simulink model "trans"  (R2017b)
settings: Solver=ode45  StartTime=0.0  StopTime=20000  RelTol=1e-3
undefined symbols (not defined in the file): dQg, dTzew, L11, L12, L21, L22, M, t0, Tg0, Twew0
settings Model: Creator=mehow  LastModifiedBy=kajaczekmackbookpro
settings DataIOCC: LimitDataPoints=on  SaveFormat=Array  SignalLoggingSaveFormat=ModelDataLogs
settings OptimizationCC: BlockReduction=off  BooleanDataType=off  LifeSpan=inf
settings DebuggingCC: SaveWithParameterizedLinksMsg=none  UnderspecifiedInitializationDetection=Classic  MergeDetectMultiDrivingBlocksExec=none  SignalResolutionControl=TryResolveAllWithWarning  MultiTaskDSMMsg=warning  MultiTaskCondExecSysMsg=none  StateNameClashWarn=warning  StrictBusMsg=None  SFUnexpectedBacktrackingDiag=warning  SFNoUnconditionalDefaultTransitionDiag=warning  SFExecutionAtInitializationDiag=none
settings HardwareCC: ProdBitPerPointer=32  ProdBitPerSizeT=32  ProdBitPerPtrDiffT=32  ProdLargestAtomicFloat=None  ProdIntDivRoundTo=Undefined  ProdEndianess=Unspecified  ProdWordSize=32  ProdHWDeviceType=32-bit Generic  TargetUnknown=on
settings ModelReferenceCC: PropagateSignalLabelsOutOfModel=off
settings CodeAppCC: StateflowObjectComments=on
settings GRTTargetCC: TargetLangStandard=C89/C90 (ANSI)  GeneratePreprocessorConditionals=Disable all
settings ConfigComp: CovMetricSettings=dw  CovHtmlReporting=on  CovSaveCumulativeToWorkspaceVar=on  CovSaveSingleToWorkspaceVar=on  CovExternalEMLEnable=off

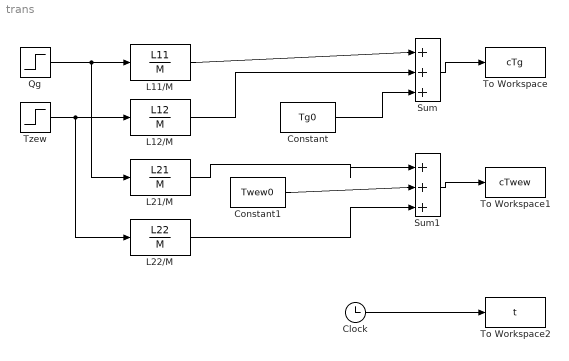
== system trans ==
  Clock : Clock
  Constant : Constant  Value=Tg0
  Constant1 : Constant  Value=Twew0
  L11/M : TransferFcn  Numerator=L11  Denominator=M
  L12/M : TransferFcn  Numerator=L12  Denominator=M
  L21/M : TransferFcn  Numerator=L21  Denominator=M
  "L22/M " : TransferFcn  Numerator=L22  Denominator=M
  "Qg " : Step  Time=t0  After=dQg  SampleTime=0
  Sum : Sum  Inputs=|+++
  Sum1 : Sum  Inputs=|+++
  To Workspace : ToWorkspace  VariableName=cTg  SampleTime=-1
  To Workspace1 : ToWorkspace  VariableName=cTwew  SampleTime=-1
  To Workspace2 : ToWorkspace  VariableName=t  SampleTime=-1
  "Tzew " : Step  Time=t0  After=dTzew  SampleTime=0
  wires:
  "Qg "/1 -> L21/M/1, L11/M/1
  "Tzew "/1 -> "L22/M "/1, L12/M/1
  Constant/1 -> Sum/3
  Sum/1 -> To Workspace/1
  Sum1/1 -> To Workspace1/1
  Clock/1 -> To Workspace2/1
  L21/M/1 -> Sum1/1
  Constant1/1 -> Sum1/2
  "L22/M "/1 -> Sum1/3
  L12/M/1 -> Sum/2
  L11/M/1 -> Sum/1
